simulink model "Entorno_Control_Virtual_2020"  (R2020b)
settings: Solver=VariableStepAuto  StartTime=0.0  StopTime=10  FixedStep=0.0001  MaxStep=0.001
model workspace (MAT data in the model file):
  A = 5
  Frec = 1
  a = 1
values from neighbouring files (symbols this model uses):
  PWM_sat = 8.78    [Parameters_MotorCC.m]
undefined symbols (not defined in the file or in its folder): National_Instruments, PCIe
libraries: fl_lib x28, nesl_utility x20, ee_lib x4, sldrtlib x3, simulink x2, pid_lib x2
settings Model: OrderedModelArguments=off  Creator=carlo  LastModifiedBy=carlo
settings DebuggingCC: UnconnectedInputMsg=none  UnconnectedOutputMsg=none  UnconnectedLineMsg=none
settings ModelReferenceCC: EnableRefExpFcnMdlSchedulingChecks=off

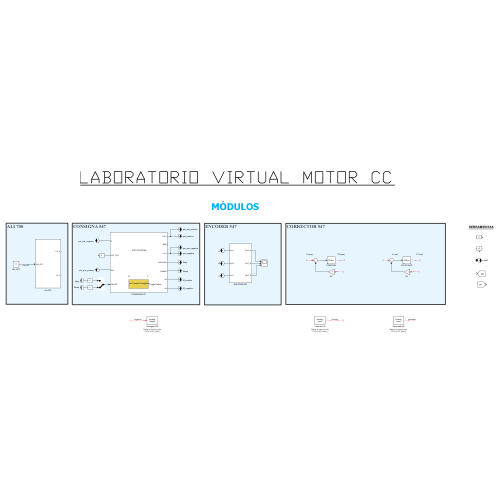
[thumbnail: Simulink's stored preview of the top-level diagram]
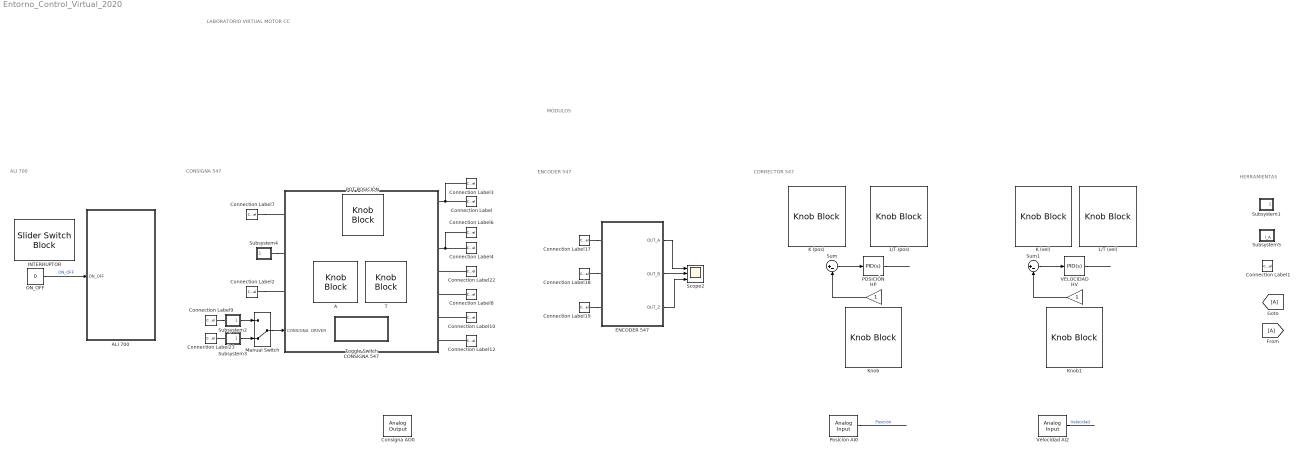
== system Entorno_Control_Virtual_2020 ==
  note: HERRAMIENTAS
  note: MÓDULOS
  note: CORRECTOR 547
  note: CONSIGNA 547
  note: ENCODER 547
  note: ALI 700
  note: LABORATORIO VIRTUAL MOTOR CC
  1/T (pos) : KnobBlock  LabelPosition=Hide  ScaleMax=10  TickInterval=1
  1/T (vel) : KnobBlock  LabelPosition=Hide  ScaleMax=10  TickInterval=1
  A : KnobBlock  LabelPosition=Hide  ScaleMax=10  TickInterval=1
  ALI 700 : Subsystem
  CONSIGNA 547 : Subsystem
      settings: PortSchema="{\"entries\":[{\"content\":{\"sides\":[{\"content\":{\"connectorIds\":[\"LConn1\",\"LConn2\",\"LConn3\",\"In1\"]},\"type\":\"ConnectorPlacement.EquallySpacedRectSide\",\"uuid\":\"4a8cfb57-dab5-486b-a591-dc2fea0d0b24\"},{\"content\":{\"connectorIds\":[\"RConn1\",\"RConn2\",\"RConn3\",\"RConn4\",\"RConn5\",\"RConn6\",\"RConn7\"],\"side\":\"RIGHT\"},\"type\":\"ConnectorPlacement.EquallySpacedRectSide\",\"uuid\":\"c23f5fb5-28b8-45c6-932c-b7e70ba2c44b\"},{\"content\":{\"side\":\"TOP\"},\"type\":\"ConnectorPlacement.EquallySpacedRectSide\",\"uuid\":\"d5136a80-57f8-4106-bad8-2d611f5e0ad7\"}]},\"type\":\"ConnectorPlacement.EquallySpacedConnector\",\"uuid\":\"b8a23e2e-242e-4702-9d69-57328d2e8c40\"}],\"packageUris\":[\"http://schema.mathworks.com/mf0/Connector/R2020b\"],\"version\":\"1.0\"}"
  Connection Label : ConnectionLabel  Label=pot_positivo
  Connection Label1 : ConnectionLabel
  Connection Label10 : ConnectionLabel  Label=M_positivo
  Connection Label12 : ConnectionLabel  Label=M_negativo
  Connection Label17 : ConnectionLabel  Label=A
  Connection Label18 : ConnectionLabel  Label=B
  Connection Label19 : ConnectionLabel  Label=Z
  Connection Label2 : ConnectionLabel  Label=pot_pos_positivo
  Connection Label22 : ConnectionLabel  Label=Step
  Connection Label23 : ConnectionLabel  Label=Ramp
  Connection Label3 : ConnectionLabel  Label=pot_pos_positivo
  Connection Label4 : ConnectionLabel  Label=pot_negativo
  Connection Label6 : ConnectionLabel  Label=pot_pos_negativo
  Connection Label7 : ConnectionLabel  Label=pot_pos_negativo
  Connection Label8 : ConnectionLabel  Label=Ramp
  Connection Label9 : ConnectionLabel  Label=Step
  Consigna AO0 : sldrtlib/Analog Output  SampleTime=0.1  MaxMissedTicks=10  ShowMissedTicks=off  YieldWhenWaiting=off  DrvName=National_Instruments/PCIe-6321  DrvAddress=4294967295  DrvOptions=[0 0 0 0 0 0 0]  Channels=1  RangeMode=1  VoltRange=1  InitialValue=[]  FinalValue=0
      settings: AttributesFormatString=National Instruments\nPCIe-6321 [auto]
  ENCODER 547 : Subsystem
  HP : Gain
  HV : Gain
  INTERRUPTOR : SliderSwitchBlock  LabelPosition=Hide
      settings: Values={{'Off', 'On'}, [0 1]}
  K (pos) : KnobBlock  LabelPosition=Hide  ScaleMax=10  TickInterval=1
  K (vel) : KnobBlock  LabelPosition=Hide  ScaleMax=10  TickInterval=1
  Knob : KnobBlock  LabelPosition=Hide  ScaleMax=1  TickInterval=0.1
  Knob1 : KnobBlock  LabelPosition=Hide  ScaleMax=2  TickInterval=0.2
  Manual Switch : ManualSwitch  CurrentSetting=0
  ON_OFF : Constant  Value=0
  POSICIÓN : pid_lib/PID Controller  Controller=PID  Form=Parallel  TimeDomain=Continuous-time  UseExternalTs=off  SampleTime=-1  IntegratorMethod=Forward Euler  FilterMethod=Forward Euler  ControllerParametersSource=internal  P=7.3781005859375  I=2.052061716715495  D=0  N=100  UseFilter=on  TunerSelectOption=Transfer Function Based (PID Tuner App)  InitialConditionSource=internal  InitialConditionForIntegrator=0  InitialConditionForFilter=0  DifferentiatorICPrevScaledInput=0  ExternalReset=none  TrackingMode=off  Kt=1  LimitOutput=off  SatLimitsSource=internal  UpperSaturationLimit=inf  LowerSaturationLimit=-inf  LinearizeAsGain=on  AntiWindupMode=none  Kb=1  POutMin=[]  POutMax=[]  IOutMin=[]  IOutMax=[]  DOutMin=[]  DOutMax=[]  NOutMin=[]  NOutMax=[]  SumOutMin=[]  SumOutMax=[]  SaturationOutMin=[]  SaturationOutMax=[]  PParamMin=[]  PParamMax=[]  IParamMin=[]  IParamMax=[]  DParamMin=[]  DParamMax=[]  NParamMin=[]  NParamMax=[]  KbParamMin=[]  KbParamMax=[]  KtParamMin=[]  KtParamMax=[]  KbOutMin=[]  KbOutMax=[]  KtOutMin=[]  KtOutMax=[]  IntegratorOutMin=[]  IntegratorOutMax=[]  FilterOutMin=[]  FilterOutMax=[]  SumI1OutMin=[]  SumI1OutMax=[]  SumI2OutMin=[]  SumI2OutMax=[]  SumI3OutMin=[]  SumI3OutMax=[]  SumI4OutMin=[]  SumI4OutMax=[]  SumDOutMin=[]  SumDOutMax=[]  DifferentiatorOutMin=[]  DifferentiatorOutMax=[]  FilterDiffOutCoefMin=[]  FilterDiffOutCoefMax=[]  ReciprocalOutMin=[]  ReciprocalOutMax=[]  SumDenOutMin=[]  SumDenOutMax=[]  SumNumOutMin=[]  SumNumOutMax=[]  DivideOutMin=[]  DivideOutMax=[]  UdiffTsProdOutMin=[]  UdiffTsProdOutMax=[]  NTsProdOutMin=[]  NTsProdOutMax=[]  UintegralTsProdOutMin=[]  UintegralTsProdOutMax=[]  UngainTsProdOutMin=[]  UngainTsProdOutMax=[]  IntegratorContinuousStateAttributes=''  IntegratorStateMustResolveToSignalObject=off  IntegratorRTWStateStorageClass=Auto  FilterContinuousStateAttributes=''  FilterStateMustResolveToSignalObject=off  FilterRTWStateStorageClass=Auto  ParallelPVariant=InternalParameters  IdealPVariant=Disabled  IVariant=InternalParameters  DVariant=InternalParameters  IntegratorVariant=Continuous  SatVariant=Disabled  AWVariant=Passthrough  PCopyVariant=Disabled  TRVariant=Disabled  FdbkBlocksVariant=Forward  IdealPFdbkVariant=Disabled  SatFdbkVariant=Disabled  DerivativeFilterVariant=ContFilter  NVariant=InternalParameters  NCopyVariant=Disabled  FilterICVariant=InternalICsFilter  IntegratorICVariant=InternalICs  ExternalResetVariant=Disabled  TRSumVariant=Passthrough  SumFdbkVariant=Disabled  SumVariant=Sum_PID  TsampFilterVariant=InternalTs  TsampNgainVariant=Passthrough  TsampIntegralVariant=Disabled_SignalSpec  ExternalSaturationOutDataTypeStr=Inherit: Same as second input
  POT POSICIÓN : KnobBlock  LabelPosition=Hide  ScaleMax=360  TickInterval=20
  Posicion AI0 : sldrtlib/Analog Input  SampleTime=0.1  MaxMissedTicks=10  ShowMissedTicks=off  YieldWhenWaiting=off  DrvName=National_Instruments/PCIe-6321  DrvAddress=4294967295  DrvOptions=[0 0 0 0 0 0 0]  Channels=1  RangeMode=1  VoltRange=1  DataType=1
      settings: AttributesFormatString=National Instruments\nPCIe-6321 [auto]
  Scope2 : Scope  NumInputPorts=3
  Subsystem1 : Subsystem
      mask Display: disp('V');
  Subsystem2 : Subsystem
      mask Display: disp('V');
  Subsystem3 : Subsystem
      mask Display: disp('V');
  Subsystem4 : Subsystem
      mask Display: disp('V');
  Subsystem5 : Subsystem
      settings: PortSchema="{\"entries\":[{\"content\":{\"sides\":[{\"content\":{\"connectorIds\":[\"LConn1\"]},\"type\":\"ConnectorPlacement.EquallySpacedRectSide\",\"uuid\":\"5f01206e-22b9-410b-acd2-df307548d4ec\"},{\"content\":{\"connectorIds\":[\"RConn1\"],\"side\":\"RIGHT\"},\"type\":\"ConnectorPlacement.EquallySpacedRectSide\",\"uuid\":\"8e9acb11-d78e-4e8a-8f36-3c08acadde04\"},{\"content\":{\"side\":\"TOP\"},\"type\":\"ConnectorPlacement.EquallySpacedRectSide\",\"uuid\":\"00b5443d-0936-4894-9d98-e1c6e581c2ec\"},{\"content\":{\"connectorIds\":[\"Out1\"],\"side\":\"BOTTOM\"},\"type\":\"ConnectorPlacement.EquallySpacedRectSide\",\"uuid\":\"fd0e1e3c-499b-4234-81ad-1a1f6c7863b2\"}]},\"type\":\"ConnectorPlacement.EquallySpacedConnector\",\"uuid\":\"3f6111df-7811-4c91-97b5-222f2bb21be8\"}],\"packageUris\":[\"http://schema.mathworks.com/mf0/Connector/R2020b\"],\"version\":\"1.0\"}"
      mask Display: disp('A');
  Sum : Sum  Inputs=|+-
  Sum1 : Sum  Inputs=|+-
  T : KnobBlock  LabelPosition=Hide  ScaleMax=10  TickInterval=1
  Toggle Switch : Subsystem  Description=Replaced Block  mask(Replaced Block){}
      mask help: This block has been replaced with an empty subsystem because it used functionality that is unavailable in Simulink R2020b.
      mask Display: fprintf('Replaced: %s\n','CustomTuningWebBlock')
  VELOCIDAD : pid_lib/PID Controller  Controller=PID  Form=Parallel  TimeDomain=Continuous-time  UseExternalTs=off  SampleTime=-1  IntegratorMethod=Forward Euler  FilterMethod=Forward Euler  ControllerParametersSource=internal  P=0  I=1  D=0  N=100  UseFilter=on  TunerSelectOption=Transfer Function Based (PID Tuner App)  InitialConditionSource=internal  InitialConditionForIntegrator=0  InitialConditionForFilter=0  DifferentiatorICPrevScaledInput=0  ExternalReset=none  TrackingMode=off  Kt=1  LimitOutput=off  SatLimitsSource=internal  UpperSaturationLimit=inf  LowerSaturationLimit=-inf  LinearizeAsGain=on  AntiWindupMode=none  Kb=1  POutMin=[]  POutMax=[]  IOutMin=[]  IOutMax=[]  DOutMin=[]  DOutMax=[]  NOutMin=[]  NOutMax=[]  SumOutMin=[]  SumOutMax=[]  SaturationOutMin=[]  SaturationOutMax=[]  PParamMin=[]  PParamMax=[]  IParamMin=[]  IParamMax=[]  DParamMin=[]  DParamMax=[]  NParamMin=[]  NParamMax=[]  KbParamMin=[]  KbParamMax=[]  KtParamMin=[]  KtParamMax=[]  KbOutMin=[]  KbOutMax=[]  KtOutMin=[]  KtOutMax=[]  IntegratorOutMin=[]  IntegratorOutMax=[]  FilterOutMin=[]  FilterOutMax=[]  SumI1OutMin=[]  SumI1OutMax=[]  SumI2OutMin=[]  SumI2OutMax=[]  SumI3OutMin=[]  SumI3OutMax=[]  SumI4OutMin=[]  SumI4OutMax=[]  SumDOutMin=[]  SumDOutMax=[]  DifferentiatorOutMin=[]  DifferentiatorOutMax=[]  FilterDiffOutCoefMin=[]  FilterDiffOutCoefMax=[]  ReciprocalOutMin=[]  ReciprocalOutMax=[]  SumDenOutMin=[]  SumDenOutMax=[]  SumNumOutMin=[]  SumNumOutMax=[]  DivideOutMin=[]  DivideOutMax=[]  UdiffTsProdOutMin=[]  UdiffTsProdOutMax=[]  NTsProdOutMin=[]  NTsProdOutMax=[]  UintegralTsProdOutMin=[]  UintegralTsProdOutMax=[]  UngainTsProdOutMin=[]  UngainTsProdOutMax=[]  IntegratorContinuousStateAttributes=''  IntegratorStateMustResolveToSignalObject=off  IntegratorRTWStateStorageClass=Auto  FilterContinuousStateAttributes=''  FilterStateMustResolveToSignalObject=off  FilterRTWStateStorageClass=Auto  ParallelPVariant=InternalParameters  IdealPVariant=Disabled  IVariant=InternalParameters  DVariant=InternalParameters  IntegratorVariant=Continuous  SatVariant=Disabled  AWVariant=Passthrough  PCopyVariant=Disabled  TRVariant=Disabled  FdbkBlocksVariant=Forward  IdealPFdbkVariant=Disabled  SatFdbkVariant=Disabled  DerivativeFilterVariant=ContFilter  NVariant=InternalParameters  NCopyVariant=Disabled  FilterICVariant=InternalICsFilter  IntegratorICVariant=InternalICs  ExternalResetVariant=Disabled  TRSumVariant=Passthrough  SumFdbkVariant=Disabled  SumVariant=Sum_PID  TsampFilterVariant=InternalTs  TsampNgainVariant=Passthrough  TsampIntegralVariant=Disabled_SignalSpec  ExternalSaturationOutDataTypeStr=Inherit: Same as second input
  Velocidad AI2 : sldrtlib/Analog Input  SampleTime=0.01  MaxMissedTicks=10  ShowMissedTicks=off  YieldWhenWaiting=off  DrvName=National_Instruments/PCIe-6321  DrvAddress=4294967295  DrvOptions=[0 0 0 0 0 0 0]  Channels=3  RangeMode=1  VoltRange=1  DataType=1
      settings: AttributesFormatString=National Instruments\nPCIe-6321 [auto]
  wires:
  ON_OFF/1 -> ALI 700/1(ON_OFF)  "ON_OFF"
  ENCODER 547/3(OUT_Z) -> Scope2/3
  ENCODER 547/2(OUT_B) -> Scope2/2
  ? -> HP/1
  Sum/1 -> POSICIÓN/1
  POSICIÓN/1 -> ?
  ? -> Sum/1
  Sum1/1 -> VELOCIDAD/1
  VELOCIDAD/1 -> ?
  HV/1 -> Sum1/2
  HP/1 -> Sum/2
  ? -> Sum1/1
  ? -> HV/1
  ENCODER 547/1(OUT_A) -> Scope2/1
  Manual Switch/1 -> CONSIGNA 547/1(CONSIGNA  DRIVER)
  Subsystem2/1(output) -> Manual Switch/1
  Subsystem3/1(output) -> Manual Switch/2
  ? -> Consigna AO0/1  "Consigna"
  Posicion AI0/1 -> ?  "Posición"
  Velocidad AI2/1 -> ?  "Velocidad"
  connections:
  Connection Label12/LConn1 -- CONSIGNA 547/RConn7
  Connection Label/LConn1 -- Connection Label3/LConn1 -- CONSIGNA 547/RConn1
  Connection Label4/LConn1 -- Connection Label6/LConn1 -- CONSIGNA 547/RConn3
  Connection Label10/LConn1 -- CONSIGNA 547/RConn6
  Connection Label17/LConn1 -- ENCODER 547/LConn1
  Connection Label18/LConn1 -- ENCODER 547/LConn2
  Connection Label19/LConn1 -- ENCODER 547/LConn3
  Connection Label22/LConn1 -- CONSIGNA 547/RConn4
  Connection Label8/LConn1 -- CONSIGNA 547/RConn5
  Connection Label9/LConn1 -- Subsystem2/LConn1
  Subsystem3/LConn1 -- Connection Label23/LConn1
  Subsystem4/LConn1 -- CONSIGNA 547/LConn2
  Connection Label2/LConn1 -- CONSIGNA 547/LConn3
  Connection Label7/LConn1 -- CONSIGNA 547/LConn1

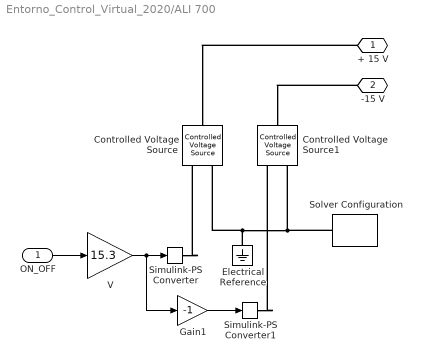
== system Entorno_Control_Virtual_2020/ALI 700 ==
  ON_OFF : Inport
  Controlled Voltage Source : fl_lib/Electrical/Electrical Sources/Controlled Voltage Source
  Controlled Voltage Source1 : fl_lib/Electrical/Electrical Sources/Controlled Voltage Source
  Electrical Reference : fl_lib/Electrical/Electrical Elements/Electrical Reference
  Gain1 : Gain  Gain=-1
  Simulink-PS Converter : nesl_utility/Simulink-PS Converter  PhysicalDomain=network_engine_domain  SubClassName=ps_input  LeftPortType=input  RightPortType=output  PseudoPeriodic=off  Frequencies=[]  NoiseDistribution=none  NoiseParameters=[]  Unit=V  AffineConversion=off  FilteringAndDerivatives=provide  SimscapeFilterOrder=1  InputFilterTimeConstant=0.001  UdotUserProvided=0
  Simulink-PS Converter1 : nesl_utility/Simulink-PS Converter  PhysicalDomain=network_engine_domain  SubClassName=ps_input  LeftPortType=input  RightPortType=output  PseudoPeriodic=off  Frequencies=[]  NoiseDistribution=none  NoiseParameters=[]  Unit=1  AffineConversion=off  FilteringAndDerivatives=provide  SimscapeFilterOrder=1  InputFilterTimeConstant=0.001  UdotUserProvided=0
  Solver Configuration : nesl_utility/Solver Configuration  PhysicalDomain=network_engine_domain  SubClassName=solver  LeftPortType=input  RightPortType=generic  Tones=[]  Harmonics=[]  SimulateNoise=off  Profile=off  UseLocalSampling=off  EnableSwitchedLinearOptims=on  FrequencyDomain=off  UseCCode=off  RelTol=0.001  AbsTol=0.001  MinStep=1e-09  ToWorkspace=off  RevertToSquareIcSolve=off  NumHomotopyIterations=100  PhasorMode=off  PhasorModeNumHarmonics=1  ConsistencySolver=NEWTON_XTOL_AFTER_FTOL  IndexReductionMethod=DerivativeReplacement  DoDC=off  ResidualTolerance=1e-09  ConsistencyTolSource=GLOBAL  ConsistencyAbsTol=0.001  ConsistencyRelTol=0.001  ConsistencyTolFactor=0.001  UseLocalSolver=off  LocalSolverChoice=NE_BACKWARD_EULER_ADVANCER  ResolveIndetEquations=on  FunctionEvalNumThread=1  LocalSolverSampleTime=0.001  DoFixedCost=off  MaxNonlinIter=3  MaxModeIter=2  ComputeImpulses=off  ImpulseIterations=2  LinearAlgebra=auto  LinearAlgebraNumThread=0  EquationFormulation=NE_TIME_EF  DelaysMemoryBudget=1024  AutomaticFiltering=on  FilteringTimeConstant=0.001  PartitionStorageMethod=AS_NEEDED  PartitionMemoryBudget=1024  PartitionMethod=ROBUST  MultibodyUseLocalSolver=off  MultibodyLocalSolverChoice=ODE1  MultibodyLocalSolverSampleTime=0.001
  V : Gain  Gain=15.3
  + 15 V : PMIOPort  Side=Right
  -15 V : PMIOPort  Port=2  Side=Right
  wires:
  ON_OFF/1 -> V/1
  Gain1/1 -> Simulink-PS Converter1/1
  V/1 -> Gain1/1, Simulink-PS Converter/1
  connections:
  Electrical Reference/LConn1 -- Solver Configuration/RConn1 -- Controlled Voltage Source1/RConn2 -- Controlled Voltage Source/RConn2
  + 15 V/RConn1 -- Controlled Voltage Source/LConn1
  -15 V/RConn1 -- Controlled Voltage Source1/LConn1
  Simulink-PS Converter/RConn1 -- Controlled Voltage Source/RConn1
  Simulink-PS Converter1/RConn1 -- Controlled Voltage Source1/RConn1

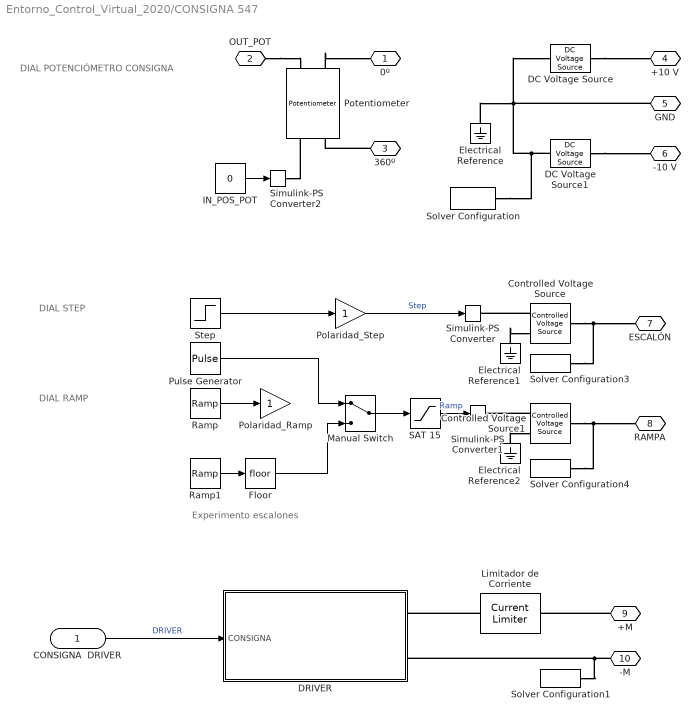
== system Entorno_Control_Virtual_2020/CONSIGNA 547 ==
  note: Experimento escalones
  note: DIAL POTENCIÓMETRO CONSIGNA
  note: DIAL STEP
  note: DIAL RAMP
  CONSIGNA  DRIVER : Inport
  Controlled Voltage Source : fl_lib/Electrical/Electrical Sources/Controlled Voltage Source
  Controlled Voltage Source1 : fl_lib/Electrical/Electrical Sources/Controlled Voltage Source
  DC Voltage Source : fl_lib/Electrical/Electrical Sources/DC Voltage Source  v0=10 V
  DC Voltage Source1 : fl_lib/Electrical/Electrical Sources/DC Voltage Source  v0=-10 V
  DRIVER : Subsystem
  Electrical Reference : fl_lib/Electrical/Electrical Elements/Electrical Reference
  Electrical Reference1 : fl_lib/Electrical/Electrical Elements/Electrical Reference
  Electrical Reference2 : fl_lib/Electrical/Electrical Elements/Electrical Reference
  Floor : Rounding
  IN_POS_POT : Constant  Value=0
  Limitador de Corriente : ee_lib/Semiconductors & Converters/Current Limiter  iLim=I_max A  vLim=0.1 V  gLim=1e-3 1/Ohm  thermal_mass=100 J/K  initial_temperature=298.15 K
      settings: InternalSimscapePortConfiguration="{\"Bottom\":[],\"Left\":[{\"id\":\"p\",\"label\":\"+\",\"type\":\"foundation.electrical.electrical\"}],\"Right\":[{\"id\":\"n\",\"label\":\"-\",\"type\":\"foundation.electrical.electrical\"}],\"Top\":[]}"
  Manual Switch : ManualSwitch
  Polaridad_Ramp : Gain
  Polaridad_Step : Gain
  Potentiometer : ee_lib/Passive/Potentiometer  nPorts=ee.enum.passive.potentiometer.nPorts.Three  R0=10 kOhm  Rw=1 Ohm  xmin=0  xmax=360  minResistance=1 Ohm  maxResistance=999 Ohm  xmin2port=0  xmax2port=1  Taper=ee.enum.passive.potentiometer.linOrLog.lin  Rcenter=200 Ohm  Gradient=ee.enum.passive.potentiometer.gradient.higherR
      settings: InternalSimscapePortConfiguration="{\"Bottom\":[],\"Left\":[{\"id\":\"pinL\",\"label\":\"L\",\"type\":\"foundation.electrical.electrical\"},{\"id\":\"W\",\"label\":\"W\",\"type\":\"foundation.electrical.electrical\"}],\"Right\":[{\"id\":\"pinR\",\"label\":\"R\",\"type\":\"foundation.electrical.electrical\"},{\"id\":\"x\",\"label\":\"x\",\"type\":\"input\"}],\"Top\":[]}"
  Pulse Generator : DiscretePulseGenerator  PulseType=Time based  Amplitude=5  Period=3  PulseWidth=50
  Ramp : simulink/Sources/Ramp  slope=0.5  start=0  InitialOutput=-10
  Ramp1 : simulink/Sources/Ramp  slope=0.125  start=0  InitialOutput=-2
  SAT 15 : Saturate  UpperLimit=15  LowerLimit=-15
  Simulink-PS Converter : nesl_utility/Simulink-PS Converter  PhysicalDomain=network_engine_domain  SubClassName=ps_input  LeftPortType=input  RightPortType=output  PseudoPeriodic=off  Frequencies=[]  NoiseDistribution=none  NoiseParameters=[]  Unit=1  AffineConversion=off  FilteringAndDerivatives=provide  SimscapeFilterOrder=1  InputFilterTimeConstant=0.001  UdotUserProvided=0
  Simulink-PS Converter1 : nesl_utility/Simulink-PS Converter  PhysicalDomain=network_engine_domain  SubClassName=ps_input  LeftPortType=input  RightPortType=output  PseudoPeriodic=off  Frequencies=[]  NoiseDistribution=none  NoiseParameters=[]  Unit=V  AffineConversion=off  FilteringAndDerivatives=provide  SimscapeFilterOrder=1  InputFilterTimeConstant=0.001  UdotUserProvided=0
  Simulink-PS Converter2 : nesl_utility/Simulink-PS Converter  PhysicalDomain=network_engine_domain  SubClassName=ps_input  LeftPortType=input  RightPortType=output  PseudoPeriodic=off  Frequencies=[]  NoiseDistribution=none  NoiseParameters=[]  Unit=1  AffineConversion=off  FilteringAndDerivatives=provide  SimscapeFilterOrder=1  InputFilterTimeConstant=0.001  UdotUserProvided=0
  Solver Configuration{,1,3..4} (4 alike) : nesl_utility/Solver Configuration  PhysicalDomain=network_engine_domain  SubClassName=solver  LeftPortType=input  RightPortType=generic  Tones=[]  Harmonics=[]  SimulateNoise=off  Profile=off  UseLocalSampling=off  EnableSwitchedLinearOptims=on  FrequencyDomain=off  UseCCode=off  RelTol=0.001  AbsTol=0.001  MinStep=1e-09  ToWorkspace=off  RevertToSquareIcSolve=off  NumHomotopyIterations=100  PhasorMode=off  PhasorModeNumHarmonics=1  ConsistencySolver=NEWTON_XTOL_AFTER_FTOL  IndexReductionMethod=DerivativeReplacement  DoDC=off  ResidualTolerance=1e-09  ConsistencyTolSource=GLOBAL  ConsistencyAbsTol=0.001  ConsistencyRelTol=0.001  ConsistencyTolFactor=0.001  UseLocalSolver=off  LocalSolverChoice=NE_BACKWARD_EULER_ADVANCER  ResolveIndetEquations=on  FunctionEvalNumThread=1  LocalSolverSampleTime=0.001  DoFixedCost=off  MaxNonlinIter=3  MaxModeIter=2  ComputeImpulses=off  ImpulseIterations=2  LinearAlgebra=auto  LinearAlgebraNumThread=0  EquationFormulation=NE_TIME_EF  DelaysMemoryBudget=1024  AutomaticFiltering=on  FilteringTimeConstant=0.001  PartitionStorageMethod=AS_NEEDED  PartitionMemoryBudget=1024  PartitionMethod=ROBUST  MultibodyUseLocalSolver=off  MultibodyLocalSolverChoice=ODE1  MultibodyLocalSolverSampleTime=0.001
  Step : Step  After=4.743883260091146  SampleTime=0
  0º : PMIOPort  Side=Left
  OUT_POT : PMIOPort  Port=2  Side=Left
  360º : PMIOPort  Port=3  Side=Left
  +10 V : PMIOPort  Port=4  Side=Right
  GND : PMIOPort  Port=5  Side=Right
  -10 V : PMIOPort  Port=6  Side=Right
  ESCALÓN : PMIOPort  Port=7  Side=Right
  RAMPA : PMIOPort  Port=8  Side=Right
  +M : PMIOPort  Port=9  Side=Right
  -M : PMIOPort  Port=10  Side=Right
  wires:
  Step/1 -> Polaridad_Step/1
  Polaridad_Step/1 -> Simulink-PS Converter/1  "Step"
  IN_POS_POT/1 -> Simulink-PS Converter2/1
  Ramp1/1 -> Floor/1
  Ramp/1 -> Polaridad_Ramp/1
  Floor/1 -> Manual Switch/2
  CONSIGNA  DRIVER/1 -> DRIVER/1(CONSIGNA)  "DRIVER"
  Manual Switch/1 -> SAT 15/1
  SAT 15/1 -> Simulink-PS Converter1/1  "Ramp"
  Pulse Generator/1 -> Manual Switch/1
  connections:
  Electrical Reference/LConn1 -- Solver Configuration/RConn1 -- DC Voltage Source1/RConn1 -- GND/RConn1 -- DC Voltage Source/RConn1
  DC Voltage Source1/LConn1 -- -10 V/RConn1
  DC Voltage Source/LConn1 -- +10 V/RConn1
  -M/RConn1 -- DRIVER/RConn2 -- Solver Configuration1/RConn1
  Simulink-PS Converter2/RConn1 -- Potentiometer/RConn2
  Potentiometer/LConn1 -- 0º/RConn1
  360º/RConn1 -- Potentiometer/RConn1
  OUT_POT/RConn1 -- Potentiometer/LConn2
  Controlled Voltage Source/RConn1 -- Simulink-PS Converter/RConn1
  Electrical Reference1/LConn1 -- Controlled Voltage Source/RConn2
  Controlled Voltage Source/LConn1 -- Solver Configuration3/RConn1 -- ESCALÓN/RConn1
  Controlled Voltage Source1/RConn1 -- Simulink-PS Converter1/RConn1
  Electrical Reference2/LConn1 -- Controlled Voltage Source1/RConn2
  Controlled Voltage Source1/LConn1 -- Solver Configuration4/RConn1 -- RAMPA/RConn1
  Limitador de Corriente/LConn1 -- DRIVER/RConn1
  +M/RConn1 -- Limitador de Corriente/RConn1

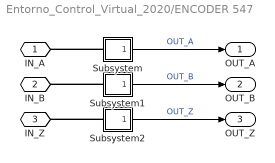
== system Entorno_Control_Virtual_2020/ENCODER 547 ==
  Subsystem : Subsystem
      mask Display: disp('V');
  Subsystem1 : Subsystem
      mask Display: disp('V');
  Subsystem2 : Subsystem
      mask Display: disp('V');
  IN_A : PMIOPort  Side=Left
  IN_B : PMIOPort  Port=2  Side=Left
  IN_Z : PMIOPort  Port=3  Side=Left
  OUT_A : Outport
  OUT_B : Outport  Port=2
  OUT_Z : Outport  Port=3
  wires:
  Subsystem2/1(output) -> OUT_Z/1  "OUT_Z"
  Subsystem1/1(output) -> OUT_B/1  "OUT_B"
  Subsystem/1(output) -> OUT_A/1  "OUT_A"
  connections:
  Subsystem/LConn1 -- IN_A/RConn1
  Subsystem1/LConn1 -- IN_B/RConn1
  Subsystem2/LConn1 -- IN_Z/RConn1

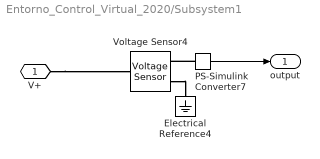
== system Entorno_Control_Virtual_2020/Subsystem1 ==
  Electrical Reference4 : fl_lib/Electrical/Electrical Elements/Electrical Reference
  PS-Simulink Converter7 : nesl_utility/PS-Simulink Converter  PhysicalDomain=network_engine_domain  SubClassName=ps_output  LeftPortType=input  RightPortType=output  PseudoPeriodic=off  Frequencies=[]  VectorFormat=inherit  Unit=V  AffineConversion=off
  Voltage Sensor4 : fl_lib/Electrical/Electrical Sensors/Voltage Sensor
  V+ : PMIOPort  Side=Left
  output : Outport
  wires:
  PS-Simulink Converter7/1 -> output/1
  connections:
  PS-Simulink Converter7/LConn1 -- Voltage Sensor4/RConn1
  Voltage Sensor4/RConn2 -- Electrical Reference4/LConn1
  V+/RConn1 -- Voltage Sensor4/LConn1

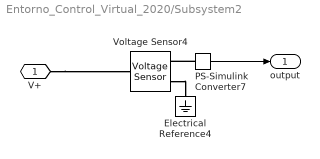
== system Entorno_Control_Virtual_2020/Subsystem2 ==
  Electrical Reference4 : fl_lib/Electrical/Electrical Elements/Electrical Reference
  PS-Simulink Converter7 : nesl_utility/PS-Simulink Converter  PhysicalDomain=network_engine_domain  SubClassName=ps_output  LeftPortType=input  RightPortType=output  PseudoPeriodic=off  Frequencies=[]  VectorFormat=inherit  Unit=V  AffineConversion=off
  Voltage Sensor4 : fl_lib/Electrical/Electrical Sensors/Voltage Sensor
  V+ : PMIOPort  Side=Left
  output : Outport
  wires:
  PS-Simulink Converter7/1 -> output/1
  connections:
  PS-Simulink Converter7/LConn1 -- Voltage Sensor4/RConn1
  Voltage Sensor4/RConn2 -- Electrical Reference4/LConn1
  V+/RConn1 -- Voltage Sensor4/LConn1

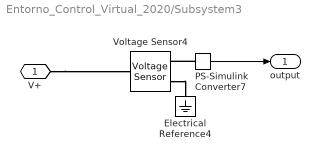
== system Entorno_Control_Virtual_2020/Subsystem3 ==
  Electrical Reference4 : fl_lib/Electrical/Electrical Elements/Electrical Reference
  PS-Simulink Converter7 : nesl_utility/PS-Simulink Converter  PhysicalDomain=network_engine_domain  SubClassName=ps_output  LeftPortType=input  RightPortType=output  PseudoPeriodic=off  Frequencies=[]  VectorFormat=inherit  Unit=V  AffineConversion=off
  Voltage Sensor4 : fl_lib/Electrical/Electrical Sensors/Voltage Sensor
  V+ : PMIOPort  Side=Left
  output : Outport
  wires:
  PS-Simulink Converter7/1 -> output/1
  connections:
  V+/RConn1 -- Voltage Sensor4/LConn1
  Voltage Sensor4/RConn2 -- Electrical Reference4/LConn1
  PS-Simulink Converter7/LConn1 -- Voltage Sensor4/RConn1

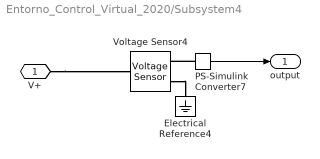
== system Entorno_Control_Virtual_2020/Subsystem4 ==
  Electrical Reference4 : fl_lib/Electrical/Electrical Elements/Electrical Reference
  PS-Simulink Converter7 : nesl_utility/PS-Simulink Converter  PhysicalDomain=network_engine_domain  SubClassName=ps_output  LeftPortType=input  RightPortType=output  PseudoPeriodic=off  Frequencies=[]  VectorFormat=inherit  Unit=V  AffineConversion=off
  Voltage Sensor4 : fl_lib/Electrical/Electrical Sensors/Voltage Sensor
  V+ : PMIOPort  Side=Left
  output : Outport
  wires:
  PS-Simulink Converter7/1 -> output/1
  connections:
  V+/RConn1 -- Voltage Sensor4/LConn1
  Voltage Sensor4/RConn2 -- Electrical Reference4/LConn1
  PS-Simulink Converter7/LConn1 -- Voltage Sensor4/RConn1

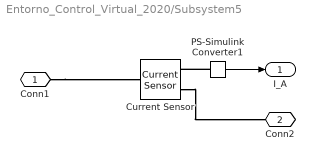
== system Entorno_Control_Virtual_2020/Subsystem5 ==
  Current Sensor : fl_lib/Electrical/Electrical Sensors/Current Sensor
  PS-Simulink Converter1 : nesl_utility/PS-Simulink Converter  PhysicalDomain=network_engine_domain  SubClassName=ps_output  LeftPortType=input  RightPortType=output  PseudoPeriodic=off  Frequencies=[]  VectorFormat=inherit  Unit=A  AffineConversion=off
  Conn1 : PMIOPort  Side=Left
  Conn2 : PMIOPort  Port=2  Side=Right
  I_A : Outport
  wires:
  PS-Simulink Converter1/1 -> I_A/1
  connections:
  PS-Simulink Converter1/LConn1 -- Current Sensor/RConn1
  Conn1/RConn1 -- Current Sensor/LConn1
  Current Sensor/RConn2 -- Conn2/RConn1

== system Entorno_Control_Virtual_2020/Toggle Switch ==

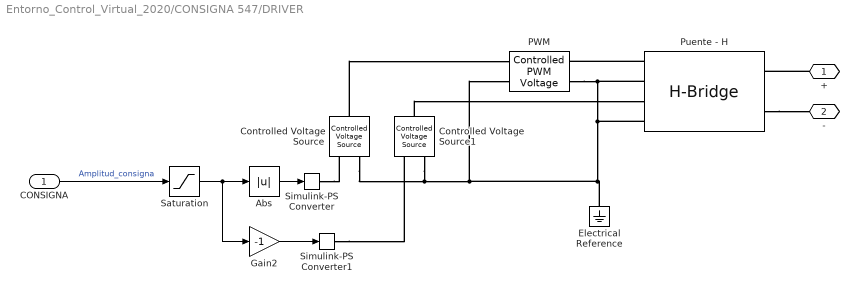
== system Entorno_Control_Virtual_2020/CONSIGNA 547/DRIVER ==
  CONSIGNA : Inport
  Abs : Abs
  Controlled Voltage Source : fl_lib/Electrical/Electrical Sources/Controlled Voltage Source
  Controlled Voltage Source1 : fl_lib/Electrical/Electrical Sources/Controlled Voltage Source
  Electrical Reference : fl_lib/Electrical/Electrical Elements/Electrical Reference
  Gain2 : Gain  Gain=-1
  PWM : ee_lib/Integrated Circuits/Controlled PWM Voltage  F=PWM_freq kHz  TD=0 s  pulse_width_offset=0 s  pulse_min=0 s  pwm_or_av=ee.enum.pwm_or_av.averaged  event_type=ee.enum.ic.event.asynchronous  sample_time=1e-6 s  Vmin=0 V  Vmax=Input_100_Duty_Cycle V  Vm=PWM_out V  u_min=0  u_max=1
  Puente - H : ee_lib/Semiconductors & Converters/Converters/H-Bridge  supply_ports=ee.enum.supply_ports.hidesupply  pwm_or_av=ee.enum.pwm_or_av.averaged  regenerative_braking_mode=ee.enum.converters.regenerative_braking_mode.depends_on_rev  discontinuous=ee.enum.current_profile.continuous  freewheeling_mode=ee.enum.converters.freewheeling_mode.one_switch_one_diode  Rload=10 Ohm  Lload=1e-5 H  F=10 kHz  Venable=2.5 V  Vmax=PWM_out V  Vreverse=0.001 V  Vbrake=2.5 V  Vm=PWM_out V  Ron=0.1 Ohm  Don=0.05 Ohm  Goff=1e-6 S  Tmeas=298.15 K  Ron2=0.1 Ohm  Don2=0.05 Ohm  Tmeas2=398.15 K  thermal_mass=100 J/K  initial_temperature=298.15 K
  Saturation : Saturate  UpperLimit=PWM_sat  LowerLimit=-PWM_sat
  Simulink-PS Converter : nesl_utility/Simulink-PS Converter  PhysicalDomain=network_engine_domain  SubClassName=ps_input  LeftPortType=input  RightPortType=output  PseudoPeriodic=off  Frequencies=[]  NoiseDistribution=none  NoiseParameters=[]  Unit=1  AffineConversion=off  FilteringAndDerivatives=provide  SimscapeFilterOrder=1  InputFilterTimeConstant=0.001  UdotUserProvided=0
  Simulink-PS Converter1 : nesl_utility/Simulink-PS Converter  PhysicalDomain=network_engine_domain  SubClassName=ps_input  LeftPortType=input  RightPortType=output  PseudoPeriodic=off  Frequencies=[]  NoiseDistribution=none  NoiseParameters=[]  Unit=1  AffineConversion=off  FilteringAndDerivatives=provide  SimscapeFilterOrder=1  InputFilterTimeConstant=0.001  UdotUserProvided=0
  + : PMIOPort  Side=Right
  - : PMIOPort  Port=2  Side=Right
  wires:
  CONSIGNA/1 -> Saturation/1  "Amplitud_consigna"
  Abs/1 -> Simulink-PS Converter/1
  Gain2/1 -> Simulink-PS Converter1/1
  Saturation/1 -> Gain2/1, Abs/1
  connections:
  Puente - H/LConn1 -- PWM/RConn1
  Controlled Voltage Source/RConn2 -- PWM/LConn2 -- Electrical Reference/LConn1 -- Puente - H/LConn4 -- PWM/RConn2 -- Puente - H/LConn2 -- Controlled Voltage Source1/RConn2
  Controlled Voltage Source1/LConn1 -- Puente - H/LConn3
  Puente - H/RConn2 -- -/RConn1
  Controlled Voltage Source/LConn1 -- PWM/LConn1
  Simulink-PS Converter/RConn1 -- Controlled Voltage Source/RConn1
  Simulink-PS Converter1/RConn1 -- Controlled Voltage Source1/RConn1
  +/RConn1 -- Puente - H/RConn1

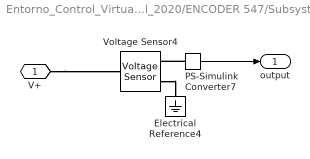
== system Entorno_Control_Virtual_2020/ENCODER 547/Subsystem ==
  Electrical Reference4 : fl_lib/Electrical/Electrical Elements/Electrical Reference
  PS-Simulink Converter7 : nesl_utility/PS-Simulink Converter  PhysicalDomain=network_engine_domain  SubClassName=ps_output  LeftPortType=input  RightPortType=output  PseudoPeriodic=off  Frequencies=[]  VectorFormat=inherit  Unit=V  AffineConversion=off
  Voltage Sensor4 : fl_lib/Electrical/Electrical Sensors/Voltage Sensor
  V+ : PMIOPort  Side=Left
  output : Outport
  wires:
  PS-Simulink Converter7/1 -> output/1
  connections:
  PS-Simulink Converter7/LConn1 -- Voltage Sensor4/RConn1
  Voltage Sensor4/RConn2 -- Electrical Reference4/LConn1
  V+/RConn1 -- Voltage Sensor4/LConn1

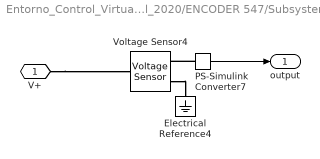
== system Entorno_Control_Virtual_2020/ENCODER 547/Subsystem1 ==
  Electrical Reference4 : fl_lib/Electrical/Electrical Elements/Electrical Reference
  PS-Simulink Converter7 : nesl_utility/PS-Simulink Converter  PhysicalDomain=network_engine_domain  SubClassName=ps_output  LeftPortType=input  RightPortType=output  PseudoPeriodic=off  Frequencies=[]  VectorFormat=inherit  Unit=V  AffineConversion=off
  Voltage Sensor4 : fl_lib/Electrical/Electrical Sensors/Voltage Sensor
  V+ : PMIOPort  Side=Left
  output : Outport
  wires:
  PS-Simulink Converter7/1 -> output/1
  connections:
  PS-Simulink Converter7/LConn1 -- Voltage Sensor4/RConn1
  Voltage Sensor4/RConn2 -- Electrical Reference4/LConn1
  V+/RConn1 -- Voltage Sensor4/LConn1

== system Entorno_Control_Virtual_2020/ENCODER 547/Subsystem2 ==
  Electrical Reference4 : fl_lib/Electrical/Electrical Elements/Electrical Reference
  PS-Simulink Converter7 : nesl_utility/PS-Simulink Converter  PhysicalDomain=network_engine_domain  SubClassName=ps_output  LeftPortType=input  RightPortType=output  PseudoPeriodic=off  Frequencies=[]  VectorFormat=inherit  Unit=V  AffineConversion=off
  Voltage Sensor4 : fl_lib/Electrical/Electrical Sensors/Voltage Sensor
  V+ : PMIOPort  Side=Left
  output : Outport
  wires:
  PS-Simulink Converter7/1 -> output/1
  connections:
  PS-Simulink Converter7/LConn1 -- Voltage Sensor4/RConn1
  Voltage Sensor4/RConn2 -- Electrical Reference4/LConn1
  V+/RConn1 -- Voltage Sensor4/LConn1
